simulink model "LPF"  (R2023b)
settings: Solver=VariableStepAuto  StartTime=0.0  StopTime=10.0  RelTol=1e-3
libraries: simulink x1

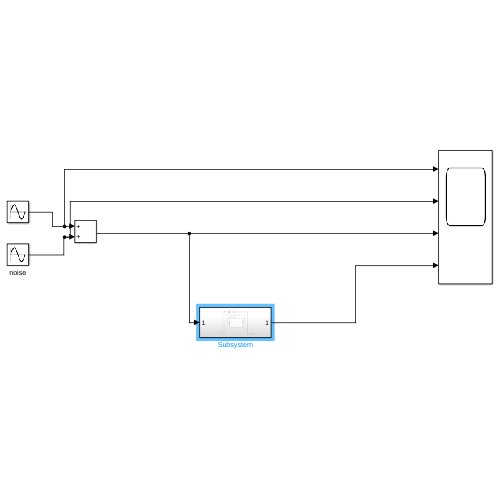
[thumbnail: Simulink's stored preview of the top-level diagram]
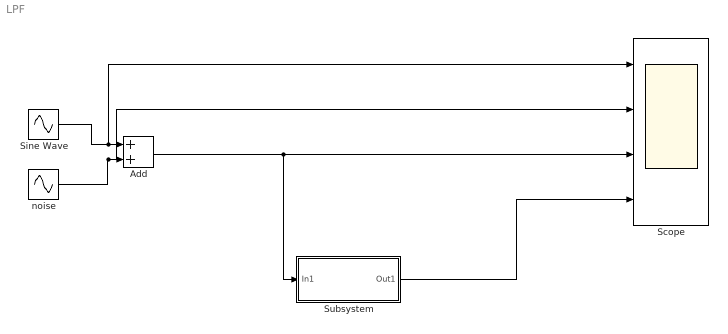
== system LPF ==
  Add : Sum
  Scope : Scope  NumInputPorts=4
  Sine Wave : Sin  SampleTime=0
  Subsystem : Subsystem
  noise : Sin  Frequency=5  SampleTime=0
  wires:
  Sine Wave/1 -> Scope/1, Add/1
  noise/1 -> Scope/2, Add/2
  Add/1 -> Subsystem/1(In1), Scope/3
  Subsystem/1(Out1) -> Scope/4

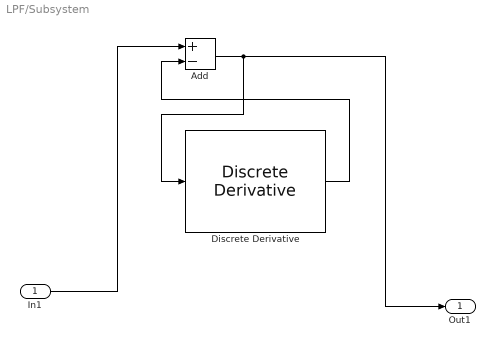
== system LPF/Subsystem ==
  In1 : Inport
  Add : Sum  Inputs=+-
  Discrete Derivative : simulink/Discrete/Discrete Derivative  gainval=1.0  ICPrevScaledInput=0.0  OutMin=[]  OutMax=[]  OutDataType=fixdt(1, 16)  OutScaling=2^-10  DoSatur=off
  Out1 : Outport
  wires:
  In1/1 -> Add/1
  Add/1 -> Discrete Derivative/1, Out1/1
  Discrete Derivative/1 -> Add/2
